simulink model "project4"  (R2025b)
settings: Solver=VariableStepAuto  StartTime=0.0  StopTime=500  RelTol=1e-3
settings Model: Creator=joefisher  LastModifiedBy=joefisher

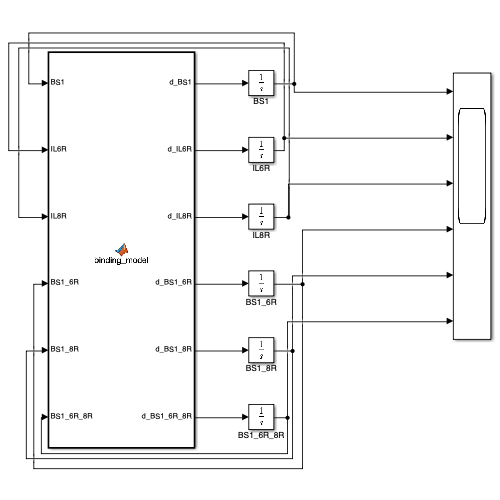
[thumbnail: Simulink's stored preview of the top-level diagram]
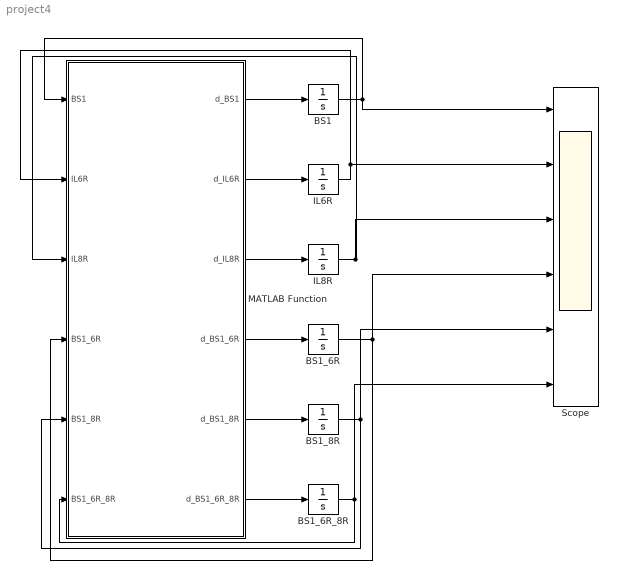
== system project4 ==
  BS1 : Integrator  InitialCondition=10
  BS1_6R : Integrator
  BS1_6R_8R : Integrator
  BS1_8R : Integrator
  IL6R : Integrator  InitialCondition=100
  IL8R : Integrator  InitialCondition=50
  MATLAB Function : MATLAB Function  TreatAsAtomicUnit=on
  Scope : Scope  NumInputPorts=6
      settings: Title=Mechanistic Binding Profile of Glofitamab Bispecific Antibody  ActiveDisplayYMinimum=-12.499999999999996  ActiveDisplayYMaximum=112.5  YLabel=Concentration (nM)
  wires:
  MATLAB Function/1(d_BS1) -> BS1/1
  MATLAB Function/2(d_IL6R) -> IL6R/1
  MATLAB Function/3(d_IL8R) -> IL8R/1
  MATLAB Function/4(d_BS1_6R) -> BS1_6R/1
  MATLAB Function/5(d_BS1_8R) -> BS1_8R/1
  MATLAB Function/6(d_BS1_6R_8R) -> BS1_6R_8R/1
  BS1/1 -> MATLAB Function/1(BS1), Scope/1
  IL6R/1 -> Scope/2, MATLAB Function/2(IL6R)
  IL8R/1 -> Scope/3, MATLAB Function/3(IL8R)
  BS1_6R/1 -> MATLAB Function/4(BS1_6R), Scope/4
  BS1_8R/1 -> MATLAB Function/5(BS1_8R), Scope/5
  BS1_6R_8R/1 -> MATLAB Function/6(BS1_6R_8R), Scope/6

== matlab function project4/MATLAB Function ==
  data: BS1 input; d_BS1 output; IL6R input; IL8R input; BS1_6R input; BS1_8R input; BS1_6R_8R input; d_IL6R output; d_IL8R output; d_BS1_6R output; d_BS1_8R output; d_BS1_6R_8R output
function [d_BS1, d_IL6R, d_IL8R, d_BS1_6R, d_BS1_8R, d_BS1_6R_8R] = binding_model(BS1, IL6R, IL8R, BS1_6R, BS1_8R, BS1_6R_8R)
    % =====================================================================
    % 1. Parameters (Glofitamab Estimates)
    % =====================================================================
    kon_BS1_6R     = 1e-4;     % On-rate for CD20
    koff_BS1_6R    = 1.6e-4;   % Off-rate for CD20
    
    kon_BS1_8R     = 1e-4;     % On-rate for CD3
    koff_BS1_8R    = 1.0e-2;   % Off-rate for CD3
    
    kon_BS1_6R_8R  = 1e-2;     % Cross-linking (CD20 arm grabbing CD3)
    koff_BS1_6R_8R = 1.0e-2;   % Cross-linking off-rate
    
    kon_BS1_8R_6R  = 1e-2;     % Cross-linking (CD3 arm grabbing CD20)
    koff_BS1_8R_6R = 1.6e-4;   % Cross-linking off-rate

    alpha = 1;                 % Volume scaling

    % =====================================================================
    % 2. Reaction Fluxes (Binding - Unbinding)
    % =====================================================================
    v_BS1_6R    = (kon_BS1_6R * BS1 * IL6R) - (koff_BS1_6R * BS1_6R);
    v_BS1_8R    = (kon_BS1_8R * BS1 * IL8R) - (koff_BS1_8R * BS1_8R);
    v_BS1_8R_6R = (kon_BS1_8R_6R * BS1_8R * IL6R) - (koff_BS1_8R_6R * BS1_6R_8R);
    v_BS1_6R_8R = (kon_BS1_6R_8R * BS1_6R * IL8R) - (koff_BS1_6R_8R * BS1_6R_8R);

    % =====================================================================
    % 3. Differential Equations (Outputs to Integrators)
    % =====================================================================
    d_BS1       = alpha * (- v_BS1_6R - v_BS1_8R);
    d_IL6R      = - v_BS1_6R - v_BS1_8R_6R;
    d_IL8R      = - v_BS1_8R - v_BS1_6R_8R;
    d_BS1_6R    = v_BS1_6R - v_BS1_6R_8R;
    d_BS1_8R    = v_BS1_8R - v_BS1_8R_6R;
    d_BS1_6R_8R = v_BS1_8R_6R + v_BS1_6R_8R;
end
